simulink model "atividade2b"  (R2024b)
settings: Solver=VariableStepAuto  StartTime=0.0  StopTime=12  RelTol=1e-3
undefined symbols (not defined in the file): A, B, DiscIntNeverNeededParam, dspblkCoreblockFVToolHelper, gcbh, kF, kGp, kr, Ts
settings Model: Creator=room2  LastModifiedBy=room2

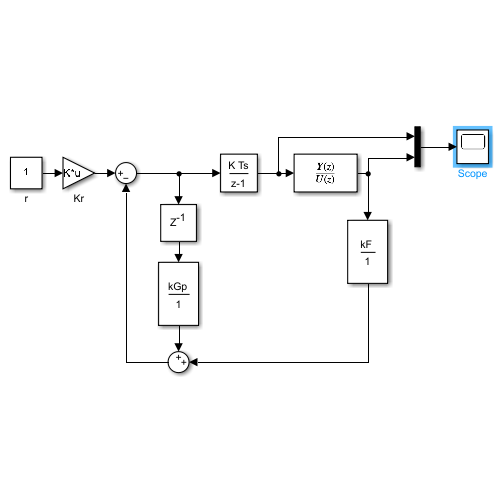
[thumbnail: Simulink's stored preview of the top-level diagram]
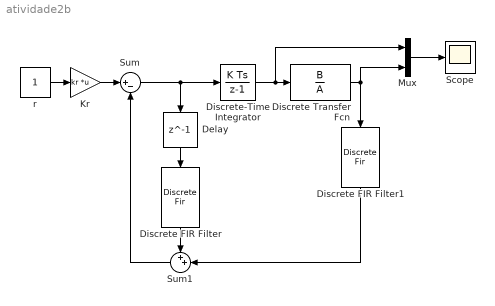
== system atividade2b ==
  Delay : Delay  DelayLength=1
  Discrete Transfer Fcn : DiscreteTransferFcn  LoadFcn=dspblkCoreblockFVToolHelper(gcbh,'load');  Numerator=B  Denominator=A
      settings: CopyFcn=dspblkCoreblockFVToolHelper(gcbh,'copy');  DeleteFcn=dspblkCoreblockFVToolHelper(gcbh,'close');  ModelCloseFcn=dspblkCoreblockFVToolHelper(gcbh,'close');  PreSaveFcn=dspblkCoreblockFVToolHelper(gcbh,'presave');  PostSaveFcn=dspblkCoreblockFVToolHelper(gcbh,'postsave');  CloseFcn=dspblkCoreblockFVToolHelper(gcbh,'close');
  Discrete FIR Filter : DiscreteFir  LoadFcn=dspblkCoreblockFVToolHelper(gcbh,'load');  Coefficients=[kGp]
      settings: CopyFcn=dspblkCoreblockFVToolHelper(gcbh,'copy');  DeleteFcn=dspblkCoreblockFVToolHelper(gcbh,'close');  ModelCloseFcn=dspblkCoreblockFVToolHelper(gcbh,'close');  PreSaveFcn=dspblkCoreblockFVToolHelper(gcbh,'presave');  PostSaveFcn=dspblkCoreblockFVToolHelper(gcbh,'postsave');  CloseFcn=dspblkCoreblockFVToolHelper(gcbh,'close');
  Discrete FIR Filter1 : DiscreteFir  LoadFcn=dspblkCoreblockFVToolHelper(gcbh,'load');  Coefficients=[kF]
      settings: CopyFcn=dspblkCoreblockFVToolHelper(gcbh,'copy');  DeleteFcn=dspblkCoreblockFVToolHelper(gcbh,'close');  ModelCloseFcn=dspblkCoreblockFVToolHelper(gcbh,'close');  PreSaveFcn=dspblkCoreblockFVToolHelper(gcbh,'presave');  PostSaveFcn=dspblkCoreblockFVToolHelper(gcbh,'postsave');  CloseFcn=dspblkCoreblockFVToolHelper(gcbh,'close');
  Discrete-Time Integrator : DiscreteIntegrator  SampleTime=Ts  ICPrevOutput=DiscIntNeverNeededParam  ICPrevScaledInput=DiscIntNeverNeededParam
  Kr : Gain  Gain=kr  Multiplication=Matrix(K*u)
  Mux : Mux  Inputs=2
  Scope : Scope
  Sum : Sum  Inputs=|+-
  Sum1 : Sum  Inputs=++|
  r : Constant
  wires:
  r/1 -> Kr/1
  Discrete Transfer Fcn/1 -> Discrete FIR Filter1/1, Mux/2
  Sum1/1 -> Sum/2
  Kr/1 -> Sum/1
  Discrete-Time Integrator/1 -> Mux/1, Discrete Transfer Fcn/1
  Mux/1 -> Scope/1
  Sum/1 -> Discrete-Time Integrator/1, Delay/1
  Delay/1 -> Discrete FIR Filter/1
  Discrete FIR Filter/1 -> Sum1/1
  Discrete FIR Filter1/1 -> Sum1/2
